simulink library "Lib_Piccolo"  (R2018b)
settings: Solver=VariableStepAuto  StartTime=0.0  StopTime=10.0  RelTol=1e-3
values from neighbouring files (symbols this model uses):
  AccelErrInt2Brakes = 0.15    [SimulationControlConfig16P.m]    (also in SimulationControlConfig16P_F0.m; SimulationControlConfig16P_F2.m; SimulationControlConfig16P_LEGACY.m; SimulationControlConfigTAILLESS.m = 0.2)
  AileronMax = 25    [SimulationControlConfig16P.m]    (also in SimulationControlConfig16P_F0.m; SimulationControlConfig16P_F2.m; SimulationControlConfig16P_LEGACY.m; SimulationControlConfigTAILLESS.m)
  AileronPower = 0.00268    [SimulationControlConfig16P.m]    (also in SimulationControlConfig16P_F0.m; SimulationControlConfig16P_F2.m; SimulationControlConfig16P_LEGACY.m; SimulationControlConfigTAILLESS.m = 0.002266)
  AileronSurfaceMax = 45    [SimulationControlConfig16P.m]    (also in SimulationControlConfig16P_F0.m; SimulationControlConfig16P_F2.m; SimulationControlConfig16P_LEGACY.m; SimulationControlConfigTAILLESS_CGAFT_F0.m = 25)
  AileronTrim = 0    [SimulationControlConfig16P.m]    (also in SimulationControlConfig16P_F0.m; SimulationControlConfig16P_F2.m; SimulationControlConfig16P_LEGACY.m; SimulationControlConfigTAILLESS.m)
  Alt = 1000 + TerrainHeight    [SimulationStateConfig.m]
  AltCruise_m = Alt * 0.3048    [SimulationControlConfig16P.m]    (also in SimulationControlConfig16P_F2.m; SimulationControlConfigTAILLESS.m = Alt/3.28084; SimulationControlConfigTAILLESS_CGAFT_F0.m = 640; SimulationControlConfigTAILLESS_CGFWD_F0.m = 640)
  AltitudeRate2PitchCmdIntegratorInit = 0.1    [SimulationControlPre.m]
  AltMax = 10000    [SimulationControlConfig16P.m]    (also in SimulationControlConfig16P_F0.m; SimulationControlConfig16P_F2.m; SimulationControlConfig16P_LEGACY.m; SimulationControlConfigTAILLESS.m)
  AltMaxAccel = 2.5    [SimulationControlConfig16P.m]    (also in SimulationControlConfig16P_F0.m = 2; SimulationControlConfig16P_F2.m = 2; SimulationControlConfig16P_LEGACY.m = 0.9; SimulationControlConfigTAILLESS.m = 2)
  AltMin = 0    [SimulationControlConfig16P.m]    (also in SimulationControlConfig16P_F0.m; SimulationControlConfig16P_F2.m; SimulationControlConfig16P_LEGACY.m; SimulationControlConfigTAILLESS.m)
  AltRateCmd2Pitch = 0.26    [SimulationControlConfig16P.m]    (also in SimulationControlConfig16P_F0.m = 0.35; SimulationControlConfig16P_F2.m = 0.35; SimulationControlConfig16P_LEGACY.m = 0.6; SimulationControlConfigTAILLESS.m = 0.9)
  AltRateError2Pitch = 0.34    [SimulationControlConfig16P.m]    (also in SimulationControlConfig16P_F0.m = 0.61; SimulationControlConfig16P_F2.m = 0.61; SimulationControlConfig16P_LEGACY.m = 0.4; SimulationControlConfigTAILLESS.m = 0.3)
  AltRateErrorInt2Pitch = 0.61    [SimulationControlConfig16P.m]    (also in SimulationControlConfig16P_F0.m = 0.28; SimulationControlConfig16P_F2.m = 0.28; SimulationControlConfig16P_LEGACY.m = 0.45; SimulationControlConfigTAILLESS.m = 0.15)
  AltRateLpfCutOff = 3    [SimulationControlConfig16P.m]    (also in SimulationControlConfig16P_F0.m; SimulationControlConfig16P_F2.m; SimulationControlConfig16P_LEGACY.m; SimulationControlConfigTAILLESS.m = 5)
  AutoNosegear2Rudder = 26    [SimulationControlConfig16P.m]    (also in SimulationControlConfig16P_F0.m; SimulationControlConfig16P_F2.m; SimulationControlConfig16P_LEGACY.m; SimulationControlConfigTAILLESS.m = 25.2)
  b = 5.54    [SimulationControlConfig16P.m]    (also in SimulationControlConfig16P_F0.m; SimulationControlConfig16P_F2.m; SimulationControlConfig16P_LEGACY.m; SimulationControlConfigTAILLESS.m = 2.37)
  Bank2AileronIntegratorInit = 0    [SimulationControlPre.m]
  BankMax_User = BankMax_User/180*pi    (= 0.610865238198)    [SimulationControlConfig16P.m]    (also in SimulationControlConfig16P_F0.m = 0.523598775598; SimulationControlConfig16P_F2.m = 0.523598775598; SimulationControlConfig16P_LEGACY.m = 0.523598775598; SimulationControlConfigTAILLESS.m = 0.558505360638)
  baseLegFlaps = 20    [SimulationControlConfig16P.m]    (also in SimulationControlConfig16P_F0.m; SimulationControlConfig16P_F2.m = 15; SimulationControlConfig16P_LEGACY.m = 0; SimulationControlConfigTAILLESS.m = 0)
  C = GeneticOpt.C    [SimulationCostFunction.m]
  c = Sw/b    (= 0.841696750903)    [SimulationControlConfig16P.m]    (also in SimulationControlConfig16P_F0.m; SimulationControlConfig16P_F2.m; SimulationControlConfig16P_LEGACY.m; SimulationControlConfigTAILLESS.m = 0.354008438819)
  cell2WheelFactorMG = 5.98    [SimulationSensorConfig16P_LEGACY.m]
  cell2WheelFactorNG = 1    [SimulationSensorConfig16P_LEGACY.m]
  cellSatMaxMG = 15000    [SimulationSensorConfig16P.m]    (also in SimulationSensorConfig16P_LEGACY.m; SimulationSensorConfigTAILLESS7P.m; SimulationSensorConfigUTAIL7P.m)
  cellSatMaxNG = 1000    [SimulationSensorConfig16P.m]    (also in SimulationSensorConfig16P_LEGACY.m; SimulationSensorConfigTAILLESS7P.m; SimulationSensorConfigUTAIL7P.m)
  cellSatMinMG = -15000    [SimulationSensorConfig16P.m]    (also in SimulationSensorConfig16P_LEGACY.m; SimulationSensorConfigTAILLESS7P.m; SimulationSensorConfigUTAIL7P.m)
  cellSatMinNG = -1000    [SimulationSensorConfig16P.m]    (also in SimulationSensorConfig16P_LEGACY.m; SimulationSensorConfigTAILLESS7P.m; SimulationSensorConfigUTAIL7P.m)
  CL_Limit = CL_Max    (= 0.54)    [SimulationControlConfig16P.m]    (also in SimulationControlConfig16P_F0.m; SimulationControlConfig16P_F2.m = 0.638; SimulationControlConfig16P_LEGACY.m; SimulationControlConfigTAILLESS.m = 0.525)
  CL_Max = 0.54    [SimulationControlConfig16P.m]    (also in SimulationControlConfig16P_F0.m; SimulationControlConfig16P_F2.m = 0.638; SimulationControlConfig16P_LEGACY.m; SimulationControlConfigTAILLESS.m = 0.525)
  CL_Max_Nom = 0.465    [SimulationControlConfig16P.m]    (also in SimulationControlConfig16P_F0.m; SimulationControlConfig16P_F2.m = 0.563; SimulationControlConfig16P_LEGACY.m; SimulationControlConfigTAILLESS.m = 0.39)
  CL_Min = 0    [SimulationControlConfig16P.m]    (also in SimulationControlConfig16P_F0.m; SimulationControlConfig16P_F2.m; SimulationControlConfig16P_LEGACY.m; SimulationControlConfigTAILLESS.m)
  ClimbMaxFraction = 0.35    [SimulationControlConfig16P.m]    (also in SimulationControlConfig16P_F0.m = 0.17; SimulationControlConfig16P_F2.m = 0.17; SimulationControlConfig16P_LEGACY.m = 0.24; SimulationControlConfigTAILLESS.m = 0.21)
  ClimboutMaxBank = 7.0    (= 7)    [SimulationControlConfig16P.m]    (also in SimulationControlConfig16P_F0.m; SimulationControlConfig16P_F2.m; SimulationControlConfig16P_LEGACY.m; SimulationControlConfigTAILLESS.m = 5)
  ClimboutTimer = 7.0    (= 7)    [SimulationControlConfig16P.m]    (also in SimulationControlConfig16P_F0.m; SimulationControlConfig16P_F2.m; SimulationControlConfig16P_LEGACY.m; SimulationControlConfigTAILLESS.m)
  dCl_per_dFlap = 0.005581818    [SimulationControlConfig16P.m]    (also in SimulationControlConfig16P_F0.m = 0; SimulationControlConfig16P_F2.m = 0.0065; SimulationControlConfig16P_LEGACY.m = 0; SimulationControlConfigTAILLESS.m = 0)
  DecelerationCmd = 3.1    [SimulationControlConfig16P.m]    (also in SimulationControlConfig16P_F0.m; SimulationControlConfig16P_F2.m; SimulationControlConfig16P_LEGACY.m; SimulationControlConfigTAILLESS.m = 0.1)
  DeRotateLogicEndTimer = abs((NoseDownLimit_Deg-1)/DeRotateRamp_Dps)    [SimulationControlConfig16P.m]    (also in SimulationControlConfig16P_F0.m; SimulationControlConfig16P_F2.m; SimulationControlConfig16P_LEGACY.m; SimulationControlConfigTAILLESS.m)
  DeRotateLogicHoldNoseUpTimer = 0.1    [SimulationControlConfig16P.m]    (also in SimulationControlConfig16P_F0.m; SimulationControlConfig16P_F2.m; SimulationControlConfig16P_LEGACY.m; SimulationControlConfigTAILLESS.m)
  DeRotateLogicTimerTimeout = 2    [SimulationControlConfig16P.m]    (also in SimulationControlConfig16P_F0.m; SimulationControlConfig16P_F2.m; SimulationControlConfig16P_LEGACY.m; SimulationControlConfigTAILLESS.m)
  DeRotateLowerCmdSaturation = 0    [SimulationControlConfig16P.m]    (also in SimulationControlConfig16P_F0.m; SimulationControlConfig16P_F2.m; SimulationControlConfig16P_LEGACY.m; SimulationControlConfigTAILLESS.m)
  DeRotateRamp_Dps = 3    [SimulationControlConfig16P.m]    (also in SimulationControlConfig16P_F0.m; SimulationControlConfig16P_F2.m; SimulationControlConfig16P_LEGACY.m; SimulationControlConfigTAILLESS.m = 8)
  DeRotateUpperCmdSaturation = 7    [SimulationControlConfig16P.m]    (also in SimulationControlConfig16P_F0.m; SimulationControlConfig16P_F2.m; SimulationControlConfig16P_LEGACY.m; SimulationControlConfigTAILLESS.m)
  DescentMaxFraction = 0.22    [SimulationControlConfig16P.m]    (also in SimulationControlConfig16P_F0.m = 0.2; SimulationControlConfig16P_F2.m = 0.2; SimulationControlConfig16P_LEGACY.m = 0.2; SimulationControlConfigTAILLESS.m = 0.17)
  DesktopSimTerrainOffset_m = 0.406    [SimulationAircraftConfig.m]
  downwindFlaps = 0    [SimulationControlConfig16P.m]    (also in SimulationControlConfig16P_F0.m; SimulationControlConfig16P_F2.m = 15; SimulationControlConfig16P_LEGACY.m; SimulationControlConfigTAILLESS.m)
  downwindSplitAil = 0    [SimulationControlConfig16P_F2.m]
  DP_init = 0.5*1.225*V_init^2    [SimulationControlConfig16P.m]    (also in SimulationControlConfig16P_F0.m; SimulationControlConfig16P_F2.m; SimulationControlConfig16P_LEGACY.m; SimulationControlConfigTAILLESS.m)
  dscNoiseMG = 1    [SimulationSensorConfig16P_LEGACY.m]
  dscNoiseNG = 0.25    [SimulationSensorConfig16P_LEGACY.m]
  DSCnumBits = 24    [SimulationSensorConfig16P.m]    (also in SimulationSensorConfig16P_LEGACY.m; SimulationSensorConfigTAILLESS7P.m; SimulationSensorConfigUTAIL7P.m)
  DSCRangeMaxMG = 15000    [SimulationSensorConfig16P.m]    (also in SimulationSensorConfig16P_LEGACY.m; SimulationSensorConfigTAILLESS7P.m; SimulationSensorConfigUTAIL7P.m)
  DSCRangeMaxNG = 1000    [SimulationSensorConfig16P.m]    (also in SimulationSensorConfig16P_LEGACY.m; SimulationSensorConfigTAILLESS7P.m; SimulationSensorConfigUTAIL7P.m)
  DSCRangeMinMG = -15000    [SimulationSensorConfig16P.m]    (also in SimulationSensorConfig16P_LEGACY.m; SimulationSensorConfigTAILLESS7P.m; SimulationSensorConfigUTAIL7P.m)
  DSCRangeMinNG = -1000    [SimulationSensorConfig16P.m]    (also in SimulationSensorConfig16P_LEGACY.m; SimulationSensorConfigTAILLESS7P.m; SimulationSensorConfigUTAIL7P.m)
  dt = DLLSim.dt    [SimulationTimeStep.m]    (also in SimulationTrim.m = 0.02)
  EarlyTouchdownThreshold = 3.0    (= 3)    [SimulationControlConfig16P.m]    (also in SimulationControlConfig16P_F0.m; SimulationControlConfig16P_F2.m; SimulationControlConfig16P_LEGACY.m; SimulationControlConfigTAILLESS.m)
  ElevatorDeflectionRate = 15    [SimulationControlConfig16P.m]    (also in SimulationControlConfig16P_F0.m; SimulationControlConfig16P_F2.m; SimulationControlConfig16P_LEGACY.m = 12; SimulationControlConfigTAILLESS.m = 5)
  ElevatorMax = 25    [SimulationControlConfig16P.m]    (also in SimulationControlConfig16P_F0.m; SimulationControlConfig16P_F2.m; SimulationControlConfig16P_LEGACY.m; SimulationControlConfigTAILLESS.m)
  ElevatorPower = -0.002209    [SimulationControlConfig16P.m]    (also in SimulationControlConfig16P_F0.m; SimulationControlConfig16P_F2.m; SimulationControlConfig16P_LEGACY.m; SimulationControlConfigTAILLESS.m = -0.002668)
  ElevatorTrim = -3.5    [SimulationControlConfig16P.m]    (also in SimulationControlConfig16P_F0.m; SimulationControlConfig16P_F2.m; SimulationControlConfig16P_LEGACY.m; SimulationControlConfigTAILLESS.m = -3)
  elevonBias = 0    [SimulationControlConfig16P.m]    (also in SimulationControlConfig16P_F0.m; SimulationControlConfig16P_F2.m; SimulationControlConfig16P_LEGACY.m; SimulationControlConfigTAILLESS.m)
  Enable_TAS_Protection = 0    [SimulationControlConfig16P.m]    (also in SimulationControlConfig16P_F0.m; SimulationControlConfig16P_F2.m; SimulationControlConfig16P_LEGACY.m; SimulationControlConfigTAILLESS.m)
  EnableCrossTrackAbort = 1    [SimulationControlConfig16P.m]    (also in SimulationControlConfigTAILLESS.m; SimulationControlConfigTAILLESS_CGAFT_F0.m; SimulationControlConfigTAILLESS_CGFWD_F0.m; SimulationControlConfigTAILLESS_CGFWD_F2.m)
  EnergyBandwidth = 0.04    [SimulationControlConfig16P.m]    (also in SimulationControlConfig16P_F0.m = 0.03; SimulationControlConfig16P_F2.m = 0.03; SimulationControlConfig16P_LEGACY.m = 0.02; SimulationControlConfigTAILLESS.m = 0.06)
  EngineLhFuelCut = 0    [SimulationAircraftConfig.m]
  EngineRhFuelCut = 0    [SimulationAircraftConfig.m]
  FastThrottleRate = 0.075    [SimulationControlConfig16P.m]    (also in SimulationControlConfig16P_F0.m = 0.05; SimulationControlConfig16P_F2.m = 0.05; SimulationControlConfig16P_LEGACY.m = 0.05; SimulationControlConfigTAILLESS.m = 0.1)
  FilterWarmUpTime = 2    [SimulationSensorConfig16P.m]    (also in SimulationSensorConfig16P_LEGACY.m; SimulationSensorConfigTAILLESS7P.m; SimulationSensorConfigUTAIL7P.m)
  finalApproachFlaps = 20    [SimulationControlConfig16P.m]    (also in SimulationControlConfig16P_F0.m; SimulationControlConfig16P_F2.m = 15; SimulationControlConfig16P_LEGACY.m = 0; SimulationControlConfigTAILLESS.m = 0)
  finalApproachSplitAil = 20    [SimulationControlConfig16P_F2.m]
  FinalDescentSlope_Deg = testPlans(testIndx).descentSlope    [SimulationControlConfig16P.m]    (also in SimulationControlConfig16P_F0.m; SimulationControlConfig16P_F2.m; SimulationControlConfig16P_LEGACY.m; SimulationControlConfigTAILLESS.m)
  flapMax = 0    [SimulationControlConfig16P.m]    (also in SimulationControlConfig16P_F0.m = 35; SimulationControlConfig16P_F2.m = 33; SimulationControlConfig16P_LEGACY.m; SimulationControlConfigTAILLESS.m)
  flapRate = 7.5    [SimulationControlConfig16P.m]    (also in SimulationControlConfig16P_F0.m; SimulationControlConfig16P_F2.m; SimulationControlConfig16P_LEGACY.m; SimulationControlConfigTAILLESS.m = 6.6)
  FlareHeight = 5    [SimulationControlConfig16P.m]    (also in SimulationControlConfig16P_F0.m; SimulationControlConfig16P_F2.m; SimulationControlConfig16P_LEGACY.m = 4.8; SimulationControlConfigTAILLESS.m = 2.75)
  FlareVerticalRate_mps = -0.4    [SimulationControlConfig16P.m]    (also in SimulationControlConfig16P_F0.m; SimulationControlConfig16P_F2.m; SimulationControlConfig16P_LEGACY.m = -0.5; SimulationControlConfigTAILLESS.m = -0.15)
  Fp_Aileron = 0.55*2*pi*RollRateLpfCutoff*dt    [SimulationControlConfig16P.m]    (also in SimulationControlConfig16P_F0.m; SimulationControlConfig16P_F2.m; SimulationControlConfig16P_LEGACY.m; SimulationControlConfigTAILLESS.m)
  Fp_Alt = 2*pi*0.55*AltBandwidth    (= 0.622035345411)    [SimulationControlConfig16P.m]    (also in SimulationControlConfig16P_F0.m; SimulationControlConfig16P_F2.m; SimulationControlConfig16P_LEGACY.m = 0.099; SimulationControlConfigTAILLESS.m = 0.207345115137)
  Fp_AltRate = 0.55*2*pi*AltRateLpfCutOff*dt    [SimulationControlConfig16P.m]    (also in SimulationControlConfig16P_F0.m; SimulationControlConfig16P_F2.m; SimulationControlConfig16P_LEGACY.m; SimulationControlConfigTAILLESS.m)
  Fp_Elevator = 0.55*2*pi*PitchRateLpfCutoff*dt    [SimulationControlConfig16P.m]    (also in SimulationControlConfig16P_F0.m; SimulationControlConfig16P_F2.m; SimulationControlConfig16P_LEGACY.m; SimulationControlConfigTAILLESS.m)
  Fp_Energy = 0.55*2*pi*EnergyBandwidth    (= 0.138230076758)    [SimulationControlConfig16P.m]    (also in SimulationControlConfig16P_F0.m = 0.103672557568; SimulationControlConfig16P_F2.m = 0.103672557568; SimulationControlConfig16P_LEGACY.m = 0.069115038379; SimulationControlConfigTAILLESS.m = 0.207345115137)
  Fp_Energy2 = 0.55*2*pi*EnergyBandwidth*dt    [SimulationControlConfig16P.m]    (also in SimulationControlConfig16P_F0.m; SimulationControlConfig16P_F2.m; SimulationControlConfig16P_LEGACY.m; SimulationControlConfigTAILLESS.m)
  Fp_Pitch = 0.55*2*pi*PitchBandwidth    (= 2.45358386245)    [SimulationControlConfig16P.m]    (also in SimulationControlConfig16P_F0.m; SimulationControlConfig16P_F2.m = 1.72787595947; SimulationControlConfig16P_LEGACY.m = 3.11017672705; SimulationControlConfigTAILLESS.m = 1.55508836353)
  Fp_Pitch_2 = 0.55*2*pi*PitchBandwidth*dt    [SimulationControlConfig16P.m]    (also in SimulationControlConfig16P_F0.m; SimulationControlConfig16P_F2.m; SimulationControlConfig16P_LEGACY.m; SimulationControlConfigTAILLESS.m)
  Fp_Roll = RollBandwidth^2    (= 1.69)    [SimulationControlConfig16P.m]    (also in SimulationControlConfig16P_F0.m = 1.44; SimulationControlConfig16P_F2.m = 1.44; SimulationControlConfig16P_LEGACY.m = 1.44; SimulationControlConfigTAILLESS.m = 1.21)
  Fp_Rudder = 0.55*2*pi*YawRateLpfCutoff*dt    [SimulationControlConfig16P.m]    (also in SimulationControlConfig16P_F0.m; SimulationControlConfig16P_F2.m; SimulationControlConfig16P_LEGACY.m; SimulationControlConfigTAILLESS.m)
  Fp_TAS = 0.55*2*pi*TASBandwidth    (= 0.103672557568)    [SimulationControlConfig16P.m]    (also in SimulationControlConfig16P_F0.m; SimulationControlConfig16P_F2.m; SimulationControlConfig16P_LEGACY.m; SimulationControlConfigTAILLESS.m = 0.172787595947)
  Fp_TAS_Filter = 2*pi*TasLpfCutoff*dt    [SimulationControlConfig16P.m]    (also in SimulationControlConfig16P_F0.m; SimulationControlConfig16P_F2.m; SimulationControlConfig16P_LEGACY.m; SimulationControlConfigTAILLESS.m)
  Fp_Turn = 0.55*2*pi*TurnErrLPFcutoff    (= 0.172787595947)    [SimulationControlConfig16P.m]    (also in SimulationControlConfig16P_F0.m = 0.0345575191895; SimulationControlConfig16P_F2.m = 0.0345575191895; SimulationControlConfig16P_LEGACY.m = 0.0345575191895; SimulationControlConfigTAILLESS.m)
  Fp_TurnDerr = 0.55*2*pi*TurnDerivativeLPFcutoff    (= 0.172787595947)    [SimulationControlConfig16P.m]    (also in SimulationControlConfig16P_F0.m = 0.0345575191895; SimulationControlConfig16P_F2.m = 0.0345575191895; SimulationControlConfig16P_LEGACY.m = 0.0345575191895; SimulationControlConfigTAILLESS.m)
  FTV = 3    [SimulationAircraftConfig.m]
  ftvStaticPositionError = 1/1.18    (= 0.847457627119)    [SimulationSensorConfig16P.m]    (also in SimulationSensorConfig16P_LEGACY.m; SimulationSensorConfigTAILLESS7P.m = 1; SimulationSensorConfigUTAIL7P.m = 1)
  g = 9.81    [SimulationStateConfig.m]
  goAroundSplitAil = 0    [SimulationControlConfig16P_F2.m]
  GustSpd_Kts = testPlans(testIndx).gustSpd    [SimulationStateConfig.m]
  GustTriggerVal = testPlans(testIndx).gustTriggerVal    [SimulationStateConfig.m]
  HeadingErr2TurnRate = 0.5    [SimulationControlConfig16P.m]    (also in SimulationControlConfig16P_F0.m; SimulationControlConfig16P_F2.m; SimulationControlConfig16P_LEGACY.m; SimulationControlConfigTAILLESS.m)
  HeadingErrDer2TurnRate = 0.3    [SimulationControlConfig16P.m]    (also in SimulationControlConfig16P_F0.m; SimulationControlConfig16P_F2.m; SimulationControlConfig16P_LEGACY.m; SimulationControlConfigTAILLESS.m)
  IASbounce = IASstall*0.8    [SimulationControlPre.m]
  IAScruiseCMD = sqrt(2*m*9.81/(1.225*Sw*CL_cruise))    [SimulationControlConfig16P.m]    (also in SimulationControlConfig16P_F0.m; SimulationControlConfig16P_F2.m; SimulationControlConfig16P_LEGACY.m; SimulationControlConfigTAILLESS.m)
  IASfinalCMD = 1.12 * IASmin    [SimulationControlConfig16P.m]    (also in SimulationControlConfig16P_F0.m = 1.14 * IASmin; SimulationControlConfig16P_F2.m = 1.10 * IASmin; SimulationControlConfig16P_LEGACY.m = 1.10 * IASmin; SimulationControlConfigTAILLESS.m = 1.14 * IASmin)
  IASflareCMD = IASstall    [SimulationControlConfig16P.m]    (also in SimulationControlConfig16P_F0.m; SimulationControlConfig16P_F2.m; SimulationControlConfig16P_LEGACY.m; SimulationControlConfigTAILLESS.m)
  IASmax = 64    [SimulationControlConfig16P.m]    (also in SimulationControlConfig16P_F0.m = 46; SimulationControlConfig16P_F2.m = 52; SimulationControlConfig16P_LEGACY.m = 46; SimulationControlConfigTAILLESS.m = 38.9)
  IASmin = sqrt(2*m*9.81/(1.225*Sw*0.9*CL_Max_Nom))    [SimulationControlConfig16P.m]    (also in SimulationControlConfig16P_F0.m; SimulationControlConfig16P_F2.m; SimulationControlConfig16P_LEGACY.m; SimulationControlConfigTAILLESS.m)
  IASshortCMD = IASstall    [SimulationControlConfig16P.m]    (also in SimulationControlConfig16P_F0.m; SimulationControlConfig16P_F2.m; SimulationControlConfig16P_LEGACY.m; SimulationControlConfigTAILLESS.m)
  IASstall = sqrt(2*m*9.81/(1.225*Sw*CL_Max))    [SimulationControlConfig16P.m]    (also in SimulationControlConfig16P_F0.m; SimulationControlConfig16P_F2.m; SimulationControlConfig16P_LEGACY.m; SimulationControlConfigTAILLESS.m)
  inFlight = 1    [SimulationControlConfig16P.m]    (also in SimulationControlConfigTAILLESS.m; SimulationControlConfigTAILLESS_CGAFT_F0.m; SimulationControlConfigTAILLESS_CGFWD_F0.m; SimulationControlConfigTAILLESS_CGFWD_F2.m)
  JetCatOffset = 5    [SimulationControlConfig16P.m]    (also in SimulationControlConfig16P_F0.m; SimulationControlConfig16P_F2.m; SimulationControlConfig16P_LEGACY.m)
  LaunchRollingElevator = -1.5    [SimulationControlConfig16P.m]    (also in SimulationControlConfig16P_F0.m; SimulationControlConfig16P_F2.m = 1.25; SimulationControlConfig16P_LEGACY.m; SimulationControlConfigTAILLESS.m = 1)
  ldg_NosegearMax = 10    [SimulationControlConfig16P.m]    (also in SimulationControlConfig16P_F0.m; SimulationControlConfig16P_F2.m; SimulationControlConfig16P_LEGACY.m; SimulationControlConfigTAILLESS.m)
  ldg_TrackVyErrInt2Nosegear = 0.1250    (= 0.125)    [SimulationControlConfig16P.m]    (also in SimulationControlConfig16P_F0.m; SimulationControlConfig16P_F2.m; SimulationControlConfig16P_LEGACY.m; SimulationControlConfigTAILLESS.m = 0.00714285714286)
  ldg_TrackVyErrPro2Nosegear = 0.35    [SimulationControlConfig16P.m]    (also in SimulationControlConfig16P_F0.m; SimulationControlConfig16P_F2.m; SimulationControlConfig16P_LEGACY.m; SimulationControlConfigTAILLESS.m = 0.0546666666667)
  ldg_TrackY2Vy = 0.07    [SimulationControlConfig16P.m]    (also in SimulationControlConfig16P_F0.m; SimulationControlConfig16P_F2.m; SimulationControlConfig16P_LEGACY.m; SimulationControlConfigTAILLESS.m = 0.17)
  ldg_Vy2NosegearScalingPower = 1.075    [SimulationControlConfig16P.m]    (also in SimulationControlConfig16P_F0.m; SimulationControlConfig16P_F2.m; SimulationControlConfig16P_LEGACY.m; SimulationControlConfigTAILLESS.m = 0.6)
  ldg_Y2VyScalingPower = 0.175    [SimulationControlConfig16P.m]    (also in SimulationControlConfig16P_F0.m; SimulationControlConfig16P_F2.m; SimulationControlConfig16P_LEGACY.m; SimulationControlConfigTAILLESS.m = 0)
  ldg_YawRate2Nosegear = 0.175    [SimulationControlConfig16P.m]    (also in SimulationControlConfig16P_F0.m; SimulationControlConfig16P_F2.m; SimulationControlConfig16P_LEGACY.m; SimulationControlConfigTAILLESS.m = 0.065)
  LiftSlope = 0.064285    [SimulationControlConfig16P.m]    (also in SimulationControlConfig16P_F0.m; SimulationControlConfig16P_F2.m; SimulationControlConfig16P_LEGACY.m; SimulationControlConfigTAILLESS.m = 0.058631)
  LPFaileronInit = 0    [SimulationControlPre.m]
  LPFclestInit = 0    [SimulationControlPre.m]
  LPFenergyFFInit = 0    [SimulationControlPre.m]
  ... (+122 more)
undefined symbols (not defined in the file or in its folder): abortFlag, alphaHPF, apmDelay, BRWNOUT, CRAWOR, CRAWUR, DiscIntNeverNeededParam, DLLSim, DLLSimStep, ECOMOR, ECOMUR, Fp_Tas, GustTrigger_HeightAgl_m, IPSTAT, LCINTEG, Ldg_Persist_Time, LOWER_FLAGS, MSG_ENABLE, NoiseStd, OLDVAL, OVERRIDE_ENABLE, OVERRIDE_VALUE, REBOOT, reversionEnable, revIASMax, revIASMin, revPitchMax, revPitchMin, revPitchRateMax, revRollMax, revRollRateMax, SAMPLE, SCALON, SensorModel, sigbuilder_block, Sim_Vx, Sim_Vy, Sim_Vz, Sim_Xpos, Sim_Ypos, Sim_Zpos, SYSOR, SYSUR, TARE, TEMPOR, TEMPUR, testIndx, testPlan, testPlans, Trim_piccoloInCmd, Trim_REFSI_FD_IN_nmodeCgShifterCmd_Flag, Trim_REFSI_FD_IN_nmodeCgShifterCmd_Ft, Trim_REFSI_FD_IN_nmodeCgShifterCmdType, Trim_REFSI_FD_IN_nmodeCgShifterNRCActive, Trim_REFSI_FD_IN_nmodeFlapLhIBCmd_Deg, Trim_REFSI_FD_IN_nmodeFlapLhOBCmd_Deg, Trim_REFSI_FD_IN_nmodeFlapRhIBCmd_Deg, Trim_REFSI_FD_IN_nmodeFlapRhOBCmd_Deg, Trim_REFSI_FD_IN_nmodeSlatLhCmd_Deg ... (+11)
libraries: simulink x1237, $bdroot x179, aerolibconvert2 x63, dspswit3 x25, aerolibatmos2 x5, simulink_extras x4, dsparch4 x2, Lib_Piccolo_Alt x2, eeGeneralControl x1, dspindex x1
(part 74 of 74)

== matlab function Lib_Piccolo/Control Allocation/M2 Flaperon and FTD/Surface Mixing Function ==
  data: Pic_AileronCmd input; PrtAileronUpperCmd output; Pic_ElevatorCmd input; PrtAileronLowerCmd output; StbdAileronUpperCmd output; StbdAileronLowerCmd output; PrtInbElevonCmd output; StbdInbdElevonCmd output; PrtOutElevonCmd output; StbdOutdElevonCmd output; ElevatorUtailCmd output; AftFlapCmd output; Pic_RudderCmd input; PylonRudderCmd output; WingletRudderCmd output; UTailRudderCmd output; Pic_FlapCmd input
function [PrtAileronUpperCmd, PrtAileronLowerCmd, StbdAileronUpperCmd, StbdAileronLowerCmd,...
          PrtInbElevonCmd, StbdInbdElevonCmd, PrtOutElevonCmd, StbdOutdElevonCmd,...
          ElevatorUtailCmd, AftFlapCmd,...
          PylonRudderCmd, WingletRudderCmd, UTailRudderCmd]= fcn(Pic_AileronCmd, Pic_ElevatorCmd, Pic_RudderCmd, Pic_FlapCmd)
    
      % Split Ailerons from flap command
      PrtAileronUpperCmd = max(-2 * Pic_FlapCmd + Pic_AileronCmd, -45);
      PrtAileronLowerCmd =  min(2 * Pic_FlapCmd + Pic_AileronCmd, 45);

      StbdAileronUpperCmd =  min(2 * Pic_FlapCmd + Pic_AileronCmd, 45);
      StbdAileronLowerCmd = max(-2 * Pic_FlapCmd + Pic_AileronCmd, -45);
      
      % Mix elevons as flaperons
      PrtInbElevonCmd   = min(Pic_AileronCmd + Pic_FlapCmd, 25);
      StbdInbdElevonCmd = min(-1*Pic_AileronCmd + Pic_FlapCmd, 25);
      
      PrtOutElevonCmd   = min(Pic_AileronCmd + Pic_FlapCmd, 25);
      StbdOutdElevonCmd = min(-1*Pic_AileronCmd + Pic_FlapCmd, 25);
      
      ElevatorUtailCmd = Pic_ElevatorCmd;
      AftFlapCmd = Pic_ElevatorCmd; 
      
      PylonRudderCmd   = Pic_RudderCmd;
      
      WingletRudderCmd = Pic_RudderCmd;
      
      UTailRudderCmd   = Pic_RudderCmd;      
end

== matlab function Lib_Piccolo/Control Allocation/M2 Flap-to-Drag 2/Surface Mixing Function ==
  data: Pic_AileronCmd input; PrtAileronUpperCmd output; Pic_ElevatorCmd input; PrtAileronLowerCmd output; StbdAileronUpperCmd output; StbdAileronLowerCmd output; PrtInbElevonCmd output; StbdInbdElevonCmd output; PrtOutElevonCmd output; StbdOutdElevonCmd output; ElevatorUtailCmd output; AftFlapCmd output; Pic_RudderCmd input; PylonRudderCmd output; WingletRudderCmd output; UTailRudderCmd output; Pic_FlapCmd input; elevonBias input; AileronMax input
function [PrtAileronUpperCmd, PrtAileronLowerCmd, StbdAileronUpperCmd, StbdAileronLowerCmd,...
          PrtInbElevonCmd, StbdInbdElevonCmd, PrtOutElevonCmd, StbdOutdElevonCmd,...
          ElevatorUtailCmd, AftFlapCmd,...
          PylonRudderCmd, WingletRudderCmd, UTailRudderCmd]= fcn(Pic_AileronCmd, Pic_ElevatorCmd, Pic_RudderCmd, Pic_FlapCmd, elevonBias, AileronMax)
    
      %Roll saturation limits
      if(Pic_AileronCmd > AileronMax)
          Pic_AileronCmd = AileronMax;
      elseif(Pic_AileronCmd < -1*AileronMax)
          Pic_AileronCmd = -1*AileronMax;
      end
      
      % If not commanding flaps, mix ailerons together
      if(Pic_FlapCmd < 0.1)
          PrtAileronUpperCmd = Pic_AileronCmd;
          PrtAileronLowerCmd = Pic_AileronCmd;

          StbdAileronUpperCmd = Pic_AileronCmd;
          StbdAileronLowerCmd = Pic_AileronCmd;
          
      % Else, mix to split ailerons
      else
          PrtAileronUpperCmd = -1 * Pic_FlapCmd + Pic_AileronCmd;
          PrtAileronLowerCmd = Pic_FlapCmd + Pic_AileronCmd;
          
          StbdAileronUpperCmd = Pic_FlapCmd + Pic_AileronCmd;
          StbdAileronLowerCmd = -1 * Pic_FlapCmd + Pic_AileronCmd;
          
          %If top or bottom aileron becomes saturated, prioritize roll authority
          if(PrtAileronUpperCmd <= -1*AileronMax)
              PrtAileronLowerCmd = 2*Pic_AileronCmd+AileronMax;
              PrtAileronUpperCmd = -1*AileronMax;
              StbdAileronUpperCmd = PrtAileronLowerCmd;
              StbdAileronLowerCmd = PrtAileronUpperCmd;
          elseif(PrtAileronLowerCmd >= AileronMax)
              PrtAileronUpperCmd = 2*Pic_AileronCmd-AileronMax;
              PrtAileronLowerCmd = AileronMax;
              StbdAileronUpperCmd = PrtAileronLowerCmd;
              StbdAileronLowerCmd = PrtAileronUpperCmd;
          end
      end
      
      PrtInbElevonCmd   = Pic_AileronCmd;
      StbdInbdElevonCmd = Pic_AileronCmd;
      
      PrtOutElevonCmd   = PrtInbElevonCmd;
      StbdOutdElevonCmd = StbdInbdElevonCmd;  
      
      % Bias elevons on split-Aileron deployment
      if(Pic_FlapCmd > 15.5)
        PrtInbElevonCmd = PrtInbElevonCmd + elevonBias; 
        PrtOutElevonCmd = PrtOutElevonCmd + elevonBias;
        
        StbdInbdElevonCmd = StbdInbdElevonCmd - elevonBias;
        StbdOutdElevonCmd = StbdOutdElevonCmd - elevonBias;
      end
        
      ElevatorUtailCmd = Pic_ElevatorCmd;
      AftFlapCmd = Pic_ElevatorCmd; 
      
      PylonRudderCmd   = Pic_RudderCmd;
      
      WingletRudderCmd = Pic_RudderCmd;
      
      UTailRudderCmd   = Pic_RudderCmd;      
end

== matlab function Lib_Piccolo/Control Allocation/M8/Surface Mixing Function ==
  data: Pic_AileronCmd input; PrtAileronUpperCmd output; Pic_ElevatorCmd input; PrtAileronLowerCmd output; StbdAileronUpperCmd output; StbdAileronLowerCmd output; PrtInbElevonCmd output; StbdInbdElevonCmd output; PrtOutElevonCmd output; StbdOutdElevonCmd output; ElevatorUtailCmd output; AftFlapCmd output; Pic_RudderCmd input; PylonRudderCmd output; WingletRudderCmd output; UTailRudderCmd output
function [PrtAileronUpperCmd, PrtAileronLowerCmd, StbdAileronUpperCmd, StbdAileronLowerCmd,...
          PrtInbElevonCmd, StbdInbdElevonCmd, PrtOutElevonCmd, StbdOutdElevonCmd,...
          ElevatorUtailCmd, AftFlapCmd,...
          PylonRudderCmd, WingletRudderCmd, UTailRudderCmd]= fcn(Pic_AileronCmd, Pic_ElevatorCmd, Pic_RudderCmd)

      PrtAileronUpperCmd = Pic_AileronCmd;
      PrtAileronLowerCmd = Pic_AileronCmd;
      
      StbdAileronUpperCmd = (-1)*Pic_AileronCmd;
      StbdAileronLowerCmd = (-1)*Pic_AileronCmd;
      
      PrtInbElevonCmd   = max(Pic_AileronCmd + Pic_ElevatorCmd);
      StbdInbdElevonCmd = max((-1)*Pic_AileronCmd + Pic_ElevatorCmd);
      
      PrtOutElevonCmd   = max(Pic_AileronCmd + Pic_ElevatorCmd);
      StbdOutdElevonCmd = max((-1)*Pic_AileronCmd + Pic_ElevatorCmd);
      
      ElevatorUtailCmd = 0;
      AftFlapCmd = Pic_ElevatorCmd; 
      
      PylonRudderCmd   = Pic_RudderCmd;
      
      WingletRudderCmd = Pic_RudderCmd;
            
      UTailRudderCmd   = 0;      
end

== matlab function Lib_Piccolo/Pitch to Elevator/Reference Frame Conversion and Pitch Rate Limit Determination/AeroVsStruct_Limit/Load Factors (nMax,nMin) at current conditions  ==
  data: Q input; nMax output; Sw input; CL_Limit input; CL_Min input; m input; nMax_User input; nMin_User input; nMin output
function [nMax, nMin] = fcn(Q, Sw, CL_Limit,CL_Min, m, nMax_User, nMin_User)

nAero_Max=Sw*Q*CL_Limit/(m*9.81);
nAero_Min=Sw*Q*CL_Min/(m*9.81);
nMax=min(nMax_User,nAero_Max);
nMin=max(nMin_User, nAero_Min);
end

== matlab function Lib_Piccolo/Pitch to Elevator/Reference Frame Conversion and Pitch Rate Limit Determination/MATLAB Function ==
  data: PitchCmd_Euler input; PitchCmd_Body output; Pitch_Euler input; Roll_Euler input; Pitch_Body output; Scalar output; PitchRateCmd_Body output; PitchRateLimit_Max output; PitchRateLimit_Min output; V input; nMax input; nMin input; PitchRateMax_User input; nPrime_Max output; nPrime_Min output
function [PitchCmd_Body,Pitch_Body, Scalar, PitchRateCmd_Body, PitchRateLimit_Max, PitchRateLimit_Min,nPrime_Max,nPrime_Min] = fcn(PitchCmd_Euler, Pitch_Euler, Roll_Euler,V,nMax,nMin,PitchRateMax_User)
g=9.81;
cPhi=cos(Roll_Euler); % input should be in radian
if (0<=cPhi)&&(cPhi<0.5)
    cPhi=0.5;
elseif (0>cPhi)&&(cPhi>-0.5)
    cPhi=-0.5;
end
Scalar=1/cPhi;
PitchCmd_Body=PitchCmd_Euler*Scalar;
Pitch_Body=Pitch_Euler*Scalar;
% PitchRateCmd_Body=abs(sin(Roll_Euler))*g/(cPhi*V); 
PitchRateCmd_Body=(sin(Roll_Euler))^2*g/(cPhi*V); 
%PitchRateCmd_Body=sin(Roll_Euler)^2*g/(cPhi^2*V); 
% error in the documentation
% Wrong in the documentation !
% nPrime_Max=nMax*(1-g)*cos(Roll_Euler)*cos(Pitch_Euler); 
% nPrime_Min=nMin*(1-g)*cos(Roll_Euler)*cos(Pitch_Euler);
nPrime_Max=(nMax-1)*cos(Roll_Euler)*cos(Pitch_Euler);
nPrime_Min=(nMin-1)*cos(Roll_Euler)*cos(Pitch_Euler);

PitchRateLimit_Max=min(PitchRateCmd_Body+PitchRateMax_User, g*nPrime_Max/V);
PitchRateLimit_Min=max(PitchRateCmd_Body-PitchRateMax_User, g*nPrime_Min/V);

% PitchRateLimit_Max=PitchRateMax_User;
% PitchRateLimit_Min=-PitchRateMax_User;
% PitchRateLimit_Max=PitchRateCmd_Body+PitchRateMax_User;
% PitchRateLimit_Min=PitchRateCmd_Body-PitchRateMax_User;
end

== matlab function Lib_Piccolo/Control Allocation/M8 Flap-to-Drag/Surface Mixing Function ==
  data: Pic_AileronCmd input; PrtAileronUpperCmd output; Pic_ElevatorCmd input; PrtAileronLowerCmd output; StbdAileronUpperCmd output; StbdAileronLowerCmd output; PrtInbElevonCmd output; StbdInbdElevonCmd output; PrtOutElevonCmd output; StbdOutdElevonCmd output; ElevatorUtailCmd output; AftFlapCmd output; Pic_RudderCmd input; PylonRudderCmd output; WingletRudderCmd output; UTailRudderCmd output; Pic_FlapCmd input
function [PrtAileronUpperCmd, PrtAileronLowerCmd, StbdAileronUpperCmd, StbdAileronLowerCmd,...
          PrtInbElevonCmd, StbdInbdElevonCmd, PrtOutElevonCmd, StbdOutdElevonCmd,...
          ElevatorUtailCmd, AftFlapCmd,...
          PylonRudderCmd, WingletRudderCmd, UTailRudderCmd]= fcn(Pic_AileronCmd, Pic_ElevatorCmd, Pic_RudderCmd, Pic_FlapCmd)

      % Mixing flap commands to split ailerons
      PrtAileronUpperCmd = max(-1 * Pic_FlapCmd + Pic_AileronCmd, -45);
      PrtAileronLowerCmd =  min(Pic_FlapCmd + Pic_AileronCmd, 45);

      StbdAileronUpperCmd = min(Pic_FlapCmd + Pic_AileronCmd, 45);
      StbdAileronLowerCmd =  max(-1 * Pic_FlapCmd + Pic_AileronCmd, -45);
          
      % Pitch and Roll mixed to Elevons
      PrtInbElevonCmd   = max(Pic_AileronCmd + Pic_ElevatorCmd);
      StbdInbdElevonCmd = max((-1)*Pic_AileronCmd + Pic_ElevatorCmd);
      
      PrtOutElevonCmd   = max(Pic_AileronCmd + Pic_ElevatorCmd);
      StbdOutdElevonCmd = max((-1)*Pic_AileronCmd + Pic_ElevatorCmd);
      
      ElevatorUtailCmd = 0;
      AftFlapCmd = Pic_ElevatorCmd; 
      
      PylonRudderCmd   = Pic_RudderCmd;
      
      WingletRudderCmd = Pic_RudderCmd;
            
      UTailRudderCmd   = 0;      
end
